simulink model "actuators_lib_example"  (R2018b)
settings: Solver=VariableStepAuto  StartTime=0.0  StopTime=10.0  RelTol=1e-3
libraries: actuators_lib x2
settings Model: Creator=yannic  LastModifiedBy=yannic

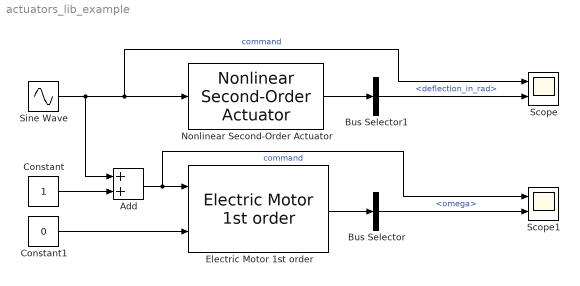
== system actuators_lib_example ==
  Add : Sum
  Bus Selector : BusSelector  OutputSignals=omega
  Bus Selector1 : BusSelector  OutputSignals=deflection_in_rad
  Constant : Constant
  Constant1 : Constant  Value=0
  Electric Motor 1st order : actuators_lib/Electric Motor 1st order  K_T=30/pi/920  J_prop=1e-04  R_i=0.042  IC_omega=0  omega_max=Inf  omega_min=0
      settings: SourceProductName=LADAC
  Nonlinear Second-Order Actuator : actuators_lib/Nonlinear Second-Order Actuator  omega=10  d=0.7  A_max=20*pi/180  A_min=-20*pi/180  dot_A_max=60*pi/180  dot_A_min=-60*pi/180  A_0=0  dot_A_0=0
      settings: SourceProductName=LADAC
  Scope : Scope  NumInputPorts=2
  Scope1 : Scope  NumInputPorts=2
  Sine Wave : Sin  SampleTime=0
  wires:
  Sine Wave/1 -> Add/1, Scope/1, Nonlinear Second-Order Actuator/1  "command"
  Add/1 -> Scope1/1, Electric Motor 1st order/1  "command"
  Constant/1 -> Add/2
  Nonlinear Second-Order Actuator/1 -> Bus Selector1/1
  Electric Motor 1st order/1 -> Bus Selector/1
  Constant1/1 -> Electric Motor 1st order/2
  Bus Selector/1 -> Scope1/2  "<omega>"
  Bus Selector1/1 -> Scope/2  "<deflection_in_rad>"
